simulink subsystem "matcher"  (R2019b)
settings: Solver=VariableStepAuto  StartTime=0.0  StopTime=10.0  RelTol=1e-3
InitFcn:
  | %% DSPBuilder Start
  | alt_dspbuilder_update_model(bdroot)
  | %% DSPBuilder End
StartFcn:
  | %% DSPBuilder Start
  | alt_dspbuilder_hdlimport_prepare_for_simulation(bdroot)
  | %% DSPBuilder End
libraries: allblocks_alteradspbuilder2 x10
settings Model: Creator=vboxuser  LastModifiedBy=vboxuser

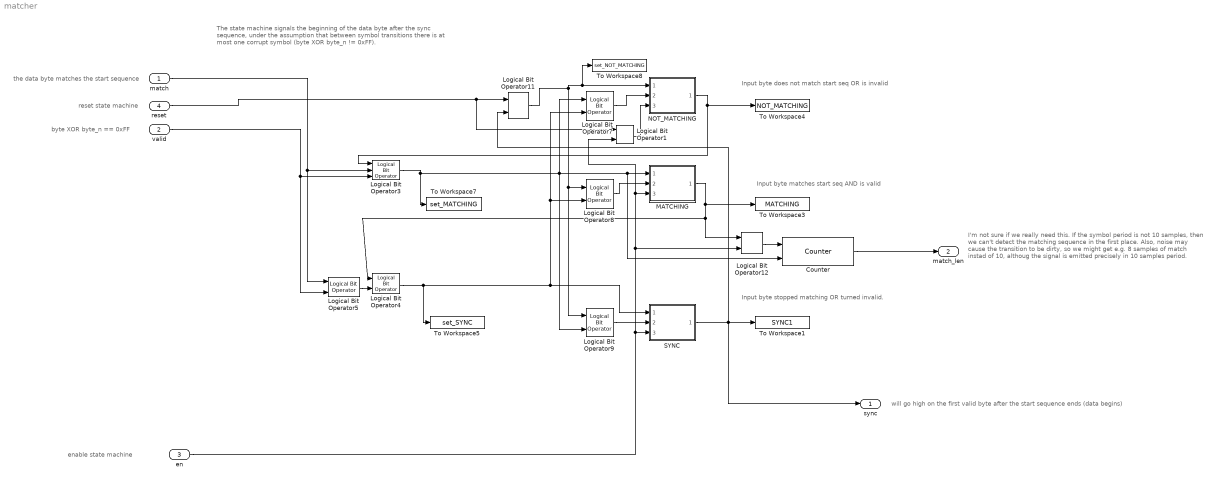
== system matcher ==
  note: I'm not sure if we really need this. If the symbol period is not 10 samples,
      | then we can't detect the matching sequence in the first place. Also, noise
      | may cause the transition to be dirty, so we might get e.g. 8 samples of
      | match instad of 10, althoug the signal is emitted precisely in 10 samples
      | period.
  note: Input byte stopped matching OR turned invalid.
  note: Input byte matches start seq AND is valid
  note: Input byte does not match start seq OR is invalid
  note: The state machine signals the beginning of the data byte after
      | the sync sequence, under the assumption that between symbol
      | transitions there is at most one corrupt symbol (byte XOR byte_n != 0xFF).
  note: will go high on the first valid byte after the start sequence ends (data begins)
  note: enable state machine
  note: byte XOR byte_n == 0xFF
  note: reset state machine
  note: the data byte matches the start sequence
  match : Inport
  valid : Inport  Port=2
  en : Inport  Port=3
  reset : Inport  Port=4
  Counter : allblocks_alteradspbuilder2/Counter  BusType=Unsigned Integer  bwl=4  bwr=0  use_modulo=off  modulo=255  SpecifyClock=off  direction=Increment  use_sload=off  use_sset=off  svalue=1  use_clk_ena=off  use_ena=on  use_sclr=on  pipeline_display=1
  Logical Bit Operator{1,7..9,11} (5 alike) : allblocks_alteradspbuilder2/Logical Bit Operator  LogicalOperator=OR  user_inputs=2  pipeline_display=0
  Logical Bit Operator12 : allblocks_alteradspbuilder2/Logical Bit Operator  LogicalOperator=AND  user_inputs=2  pipeline_display=0
  Logical Bit Operator3 : allblocks_alteradspbuilder2/Logical Bit Operator  LogicalOperator=AND  user_inputs=3  pipeline_display=0
  Logical Bit Operator4 : allblocks_alteradspbuilder2/Logical Bit Operator  LogicalOperator=AND  user_inputs=2  pipeline_display=0
  Logical Bit Operator5 : allblocks_alteradspbuilder2/Logical Bit Operator  LogicalOperator=NAND  user_inputs=2  pipeline_display=0
  MATCHING : Subsystem  ReferencedSubsystem=state
  NOT_MATCHING : Subsystem  ReferencedSubsystem=state
  SYNC : Subsystem  ReferencedSubsystem=state
  To Workspace1 : ToWorkspace  VariableName=SYNC1  SampleTime=-1
      settings: Save2DSignal=2-D array (concatenate along first dimension)
  To Workspace3 : ToWorkspace  VariableName=MATCHING  SampleTime=-1
      settings: Save2DSignal=2-D array (concatenate along first dimension)
  To Workspace4 : ToWorkspace  VariableName=NOT_MATCHING  SampleTime=-1
      settings: Save2DSignal=2-D array (concatenate along first dimension)
  To Workspace5 : ToWorkspace  VariableName=set_SYNC  SampleTime=-1
      settings: Save2DSignal=2-D array (concatenate along first dimension)
  To Workspace7 : ToWorkspace  VariableName=set_MATCHING  SampleTime=-1
      settings: Save2DSignal=2-D array (concatenate along first dimension)
  To Workspace8 : ToWorkspace  VariableName=set_NOT_MATCHING  SampleTime=-1
      settings: Save2DSignal=2-D array (concatenate along first dimension)
  sync : Outport
  match_len : Outport  Port=2
  wires:
  Logical Bit Operator11/1 -> Logical Bit Operator8/1, Logical Bit Operator9/1, NOT_MATCHING/1, To Workspace8/1
  Logical Bit Operator7/1 -> NOT_MATCHING/2
  en/1 -> SYNC/3, Logical Bit Operator12/2, MATCHING/3, Logical Bit Operator1/2
  Logical Bit Operator4/1 -> SYNC/1, Logical Bit Operator7/2, Logical Bit Operator8/2, To Workspace5/1
  Logical Bit Operator3/1 -> Logical Bit Operator9/2, Counter/2, MATCHING/1, Logical Bit Operator7/1, To Workspace7/1
  Logical Bit Operator8/1 -> MATCHING/2
  match/1 -> Logical Bit Operator3/2, Logical Bit Operator5/1
  MATCHING/1 -> To Workspace3/1, Logical Bit Operator12/1, Logical Bit Operator4/1
  Logical Bit Operator9/1 -> SYNC/2
  reset/1 -> Logical Bit Operator11/1, Logical Bit Operator1/1
  Logical Bit Operator5/1 -> Logical Bit Operator4/2
  SYNC/1 -> Logical Bit Operator11/2, sync/1, To Workspace1/1
  NOT_MATCHING/1 -> Logical Bit Operator3/1, To Workspace4/1
  valid/1 -> Logical Bit Operator3/3, Logical Bit Operator5/2
  Logical Bit Operator12/1 -> Counter/1
  Counter/1 -> match_len/1
  Logical Bit Operator1/1 -> NOT_MATCHING/3
